simulink model "Momentum_Wheel_Model"  (R2019a)
settings: Solver=FixedStepAuto  StartTime=0.0  StopTime=t  FixedStep=dt  RelTol=1e-3
values from neighbouring files (symbols this model uses):
  alpha_x = 0    [SCUBED_ADACS.m]
  alpha_y = 0    [SCUBED_ADACS.m]
  alpha_z = 0    [SCUBED_ADACS.m]
  I = 2*10^-3    (= 0.002)    [SCUBED_ADACS.m]    (also in test_case_1.m)
  J_I = A + I + 2*J    (= 0.036)    [SCUBED_ADACS.m]
  J_II = B + I + 2*J    (= 0.025)    [SCUBED_ADACS.m]
  J_III = C + I + 2*J    (= 0.05)    [SCUBED_ADACS.m]
  M_SRP = 10^-4    (= 0.0001)    [SCUBED_ADACS.m]    (also in test_case_1.m)
  Mgx = 10^-11    (= 1e-11)    [SCUBED_ADACS.m]
  Mgy = 10^-11    (= 1e-11)    [SCUBED_ADACS.m]
  Mgz = 10^-11    (= 1e-11)    [SCUBED_ADACS.m]
  omega_x = 2*pi/T_EHO    (= 1.99098659277e-07)    [SCUBED_ADACS.m]    (also in test_case_1.m)
  omega_y = 0    [SCUBED_ADACS.m]
  omega_z = 0    [SCUBED_ADACS.m]
settings Model: PauseTimes=2900000  Creator=jepar  LastModifiedBy=jepar

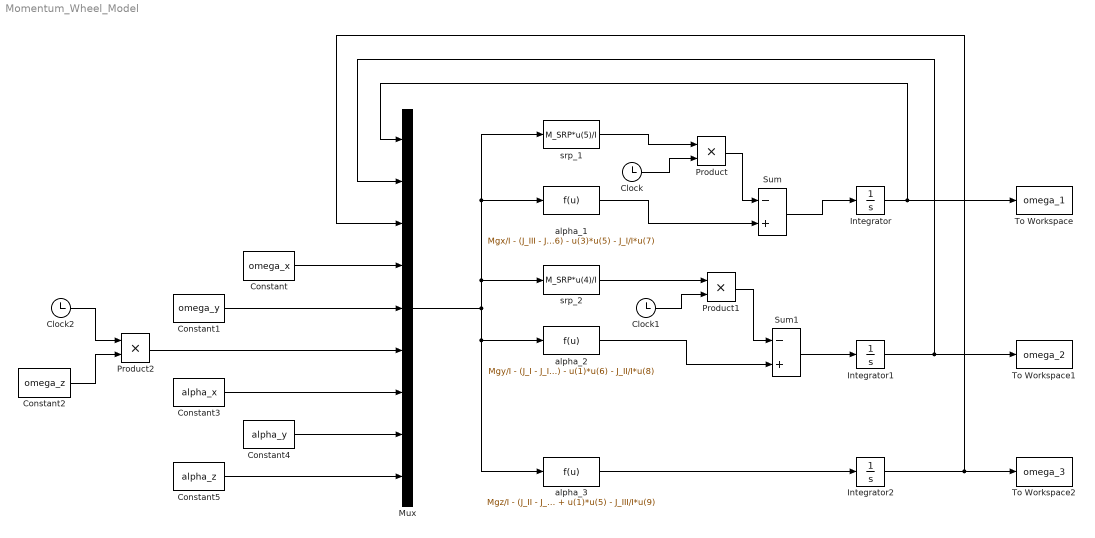
== system Momentum_Wheel_Model ==
  Clock : Clock
      settings: Decimation=clock_decimation
  Clock1 : Clock
      settings: Decimation=clock_decimation
  Clock2 : Clock
      settings: Decimation=clock_decimation
  Constant : Constant  Value=omega_x
  Constant1 : Constant  Value=omega_y
  Constant2 : Constant  Value=omega_z
  Constant3 : Constant  Value=alpha_x
  Constant4 : Constant  Value=alpha_y
  Constant5 : Constant  Value=alpha_z
  Integrator : Integrator
  Integrator1 : Integrator
  Integrator2 : Integrator
  Mux : Mux  Inputs=9
  Product : Product
  Product1 : Product
  Product2 : Product
  Sum : Sum  Inputs=-+
  Sum1 : Sum  Inputs=-+
  To Workspace : ToWorkspace  VariableName=omega_1  SaveFormat=Structure With Time  SampleTime=-1
      settings: Decimation=vector_decimation  Save2DSignal=2-D array (concatenate along first dimension)
  To Workspace1 : ToWorkspace  VariableName=omega_2  SaveFormat=Structure With Time  SampleTime=-1
      settings: Decimation=vector_decimation  Save2DSignal=2-D array (concatenate along first dimension)
  To Workspace2 : ToWorkspace  VariableName=omega_3  SaveFormat=Structure With Time  SampleTime=-1
      settings: Decimation=vector_decimation  Save2DSignal=2-D array (concatenate along first dimension)
  alpha_1 : Fcn  Expr=Mgx/I - (J_III - J_II)/I*u(5)*u(6) + u(2)*u(6) - u(3)*u(5) - J_I/I*u(7)
  alpha_2 : Fcn  Expr=Mgy/I - (J_I - J_III)/I*u(4)*u(6) + u(3)*u(4) - u(1)*u(6) - J_II/I*u(8)
  alpha_3 : Fcn  Expr=Mgz/I - (J_II - J_I)/I*u(4)*u(5) - u(2)*u(4) + u(1)*u(5) - J_III/I*u(9)
  "srp_1 " : Fcn  Expr=M_SRP*u(5)/I
  srp_2 : Fcn  Expr=M_SRP*u(4)/I
  wires:
  Integrator1/1 -> Mux/2, To Workspace1/1
  Constant3/1 -> Mux/7
  Constant4/1 -> Mux/8
  Constant5/1 -> Mux/9
  Mux/1 -> alpha_3/1, alpha_2/1, srp_2/1, "srp_1 "/1, alpha_1/1
  Integrator/1 -> To Workspace/1, Mux/1
  Integrator2/1 -> To Workspace2/1, Mux/3
  Constant1/1 -> Mux/5
  Constant/1 -> Mux/4
  alpha_1/1 -> Sum/2
  "srp_1 "/1 -> Product/1
  Clock/1 -> Product/2
  Product/1 -> Sum/1
  Sum/1 -> Integrator/1
  srp_2/1 -> Product1/1
  Clock1/1 -> Product1/2
  alpha_2/1 -> Sum1/2
  Product1/1 -> Sum1/1
  Sum1/1 -> Integrator1/1
  alpha_3/1 -> Integrator2/1
  Clock2/1 -> Product2/1
  Constant2/1 -> Product2/2
  Product2/1 -> Mux/6
